simulink model "filter_path"  (R2020b)
settings: Solver=FixedStepDiscrete  StartTime=0.0  StopTime=stopTime  FixedStep=2.0833333333333333e-05  RelTol=1e-3
settings Model: Creator=Ross  LastModifiedBy=conno
settings DataIOCC: SaveOutput=off  SaveTime=off  ReturnWorkspaceOutputs=off
settings OptimizationCC: BlockReduction=off  ConditionallyExecuteInputs=off  DefaultParameterBehavior=Inlined
settings DebuggingCC: ReadBeforeWriteMsg=DisableAll  WriteAfterWriteMsg=DisableAll  WriteAfterReadMsg=DisableAll  AlgebraicLoopMsg=error  MultiTaskDSMMsg=none  SingleTaskRateTransMsg=error  PregeneratedLibrarySubsystemCodeDiagnostic=none  ArithmeticOperatorsInVariantConditions=warning
settings HardwareCC: ProdBitPerPointer=32  ProdBitPerSizeT=32  ProdBitPerPtrDiffT=32  ProdLargestAtomicFloat=None  ProdIntDivRoundTo=Undefined  ProdEndianess=Unspecified  ProdWordSize=32  ProdHWDeviceType=ASIC/FPGA->ASIC/FPGA  TargetBitPerPointer=64  TargetBitPerSizeT=64  TargetBitPerPtrDiffT=64  TargetLongLongMode=on  TargetIntDivRoundTo=Zero  TargetEndianess=LittleEndian  TargetWordSize=64  TargetHWDeviceType=Custom Processor->MATLAB Host Computer  ProdEqTarget=off
settings ModelReferenceCC: UpdateModelReferenceTargets=IfOutOfDate  ModelReferenceNumInstancesAllowed=Single
settings SFSimCC: SFSimEcho=off  SimUseLocalCustomCode=off  CustomCodeUndefinedFunction=UseInterfaceOnly
settings RTWCC: RTWUseLocalCustomCode=off

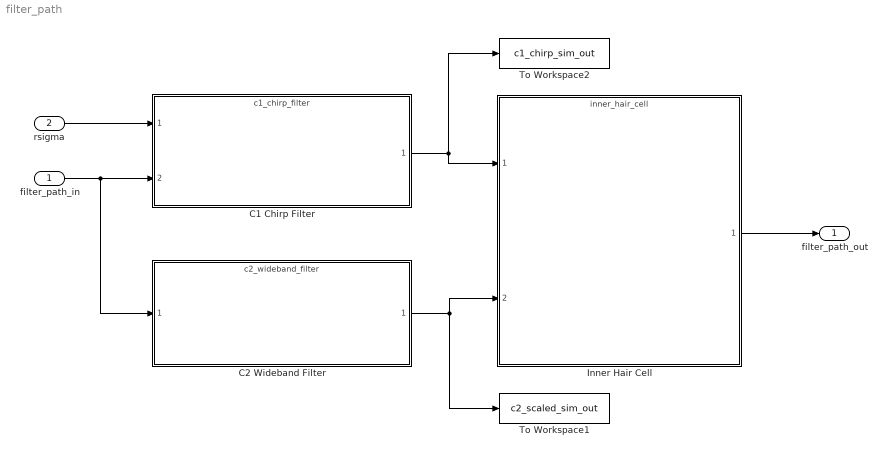
== system filter_path ==
  filter_path_in : Inport  OutDataTypeStr=single  PortDimensions=1  SampleTime=[2.0833333333333333e-05,0]
  rsigma : Inport  Port=2  OutDataTypeStr=single  PortDimensions=1  SampleTime=[2.0833333333333333e-05,0]
  C1 Chirp Filter : ModelReference  ModelNameDialog=c1_chirp_filter  SimulationMode=Normal  ModelReferenceVersion=1.135
  C2 Wideband Filter : ModelReference  ModelNameDialog=c2_wideband_filter.slx  SimulationMode=Normal  ModelReferenceVersion=1.114
  Inner Hair Cell : ModelReference  ModelNameDialog=inner_hair_cell.slx  SimulationMode=Normal  ModelReferenceVersion=1.139
  To Workspace1 : ToWorkspace  VariableName=c2_scaled_sim_out  SampleTime=-1
  To Workspace2 : ToWorkspace  VariableName=c1_chirp_sim_out  SampleTime=-1
  filter_path_out : Outport  OutDataTypeStr=single  PortDimensions=1  SampleTime=[2.0833333333333333e-05,0]
  wires:
  filter_path_in/1 -> C1 Chirp Filter/2, C2 Wideband Filter/1
  C1 Chirp Filter/1 -> To Workspace2/1, Inner Hair Cell/1
  Inner Hair Cell/1 -> filter_path_out/1
  rsigma/1 -> C1 Chirp Filter/1
  C2 Wideband Filter/1 -> To Workspace1/1, Inner Hair Cell/2
